simulink model "Week1_pr6"  (R2020b)
settings: Solver=VariableStepAuto  StartTime=0.0  StopTime=10.0  RelTol=1e-3
settings Model: Creator=user  LastModifiedBy=user

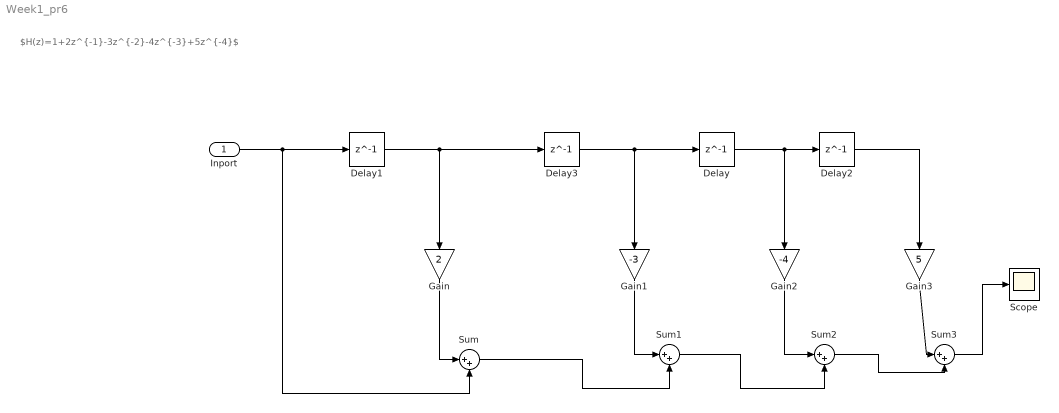
== system Week1_pr6 ==
  note: $H(z)=1+2z^{-1}-3z^{-2}-4z^{-3}+5z^{-4}$
  Inport : Inport
  Delay{,1..3} (4 alike) : Delay  DelayLength=1
  Gain : Gain  Gain=2
  Gain1 : Gain  Gain=-3
  Gain2 : Gain  Gain=-4
  Gain3 : Gain  Gain=5
  Scope : Scope
  Sum{,1..3} (4 alike) : Sum  Inputs=|++
  wires:
  Sum2/1 -> Sum3/2
  Gain3/1 -> Sum3/1
  Sum1/1 -> Sum2/2
  Sum/1 -> Sum1/2
  Delay3/1 -> Gain1/1, Delay/1
  Gain2/1 -> Sum2/1
  Delay/1 -> Gain2/1, Delay2/1
  Inport/1 -> Sum/2, Delay1/1
  Sum3/1 -> Scope/1
  Gain1/1 -> Sum1/1
  Gain/1 -> Sum/1
  Delay1/1 -> Delay3/1, Gain/1
  Delay2/1 -> Gain3/1
